simulink model "ArduinoCollectionEEGSimulation"  (R2024b)
settings: Solver=VariableStepAuto  StartTime=0.0  StopTime=10.0  RelTol=1e-3
libraries: dspfdesign x48, arduinolib x16, deeplib x16, audioai x16
settings Model: Creator=dhruva  LastModifiedBy=dhruva

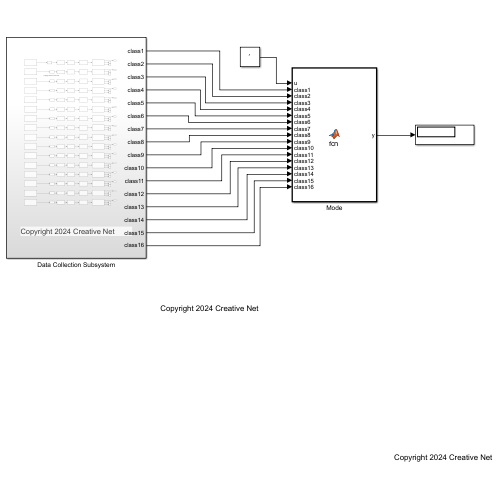
[thumbnail: Simulink's stored preview of the top-level diagram]
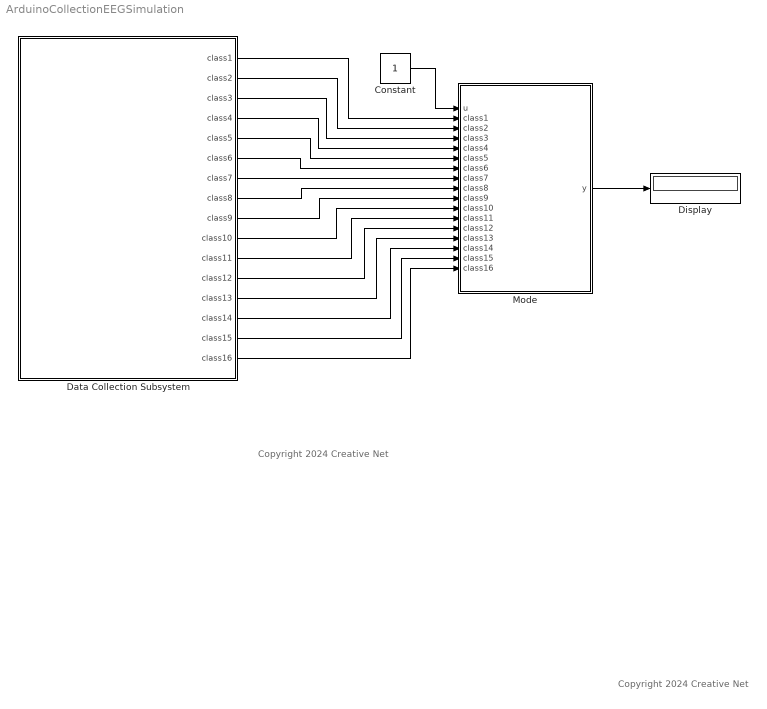
== system ArduinoCollectionEEGSimulation ==
  note: Copyright 2024 Creative Net
  note: Copyright 2024 Creative Net
  Constant : Constant
  Data Collection Subsystem : Subsystem
  Display : Display
  Mode : MATLAB Function  TreatAsAtomicUnit=on
  wires:
  Data Collection Subsystem/1(class1) -> Mode/2(class1)
  Data Collection Subsystem/2(class2) -> Mode/3(class2)
  Data Collection Subsystem/16(class16) -> Mode/17(class16)
  Data Collection Subsystem/15(class15) -> Mode/16(class15)
  Data Collection Subsystem/14(class14) -> Mode/15(class14)
  Data Collection Subsystem/13(class13) -> Mode/14(class13)
  Data Collection Subsystem/12(class12) -> Mode/13(class12)
  Data Collection Subsystem/11(class11) -> Mode/12(class11)
  Data Collection Subsystem/10(class10) -> Mode/11(class10)
  Data Collection Subsystem/3(class3) -> Mode/4(class3)
  Data Collection Subsystem/4(class4) -> Mode/5(class4)
  Data Collection Subsystem/5(class5) -> Mode/6(class5)
  Data Collection Subsystem/6(class6) -> Mode/7(class6)
  Data Collection Subsystem/7(class7) -> Mode/8(class7)
  Data Collection Subsystem/8(class8) -> Mode/9(class8)
  Data Collection Subsystem/9(class9) -> Mode/10(class9)
  Constant/1 -> Mode/1(u)
  Mode/1(y) -> Display/1

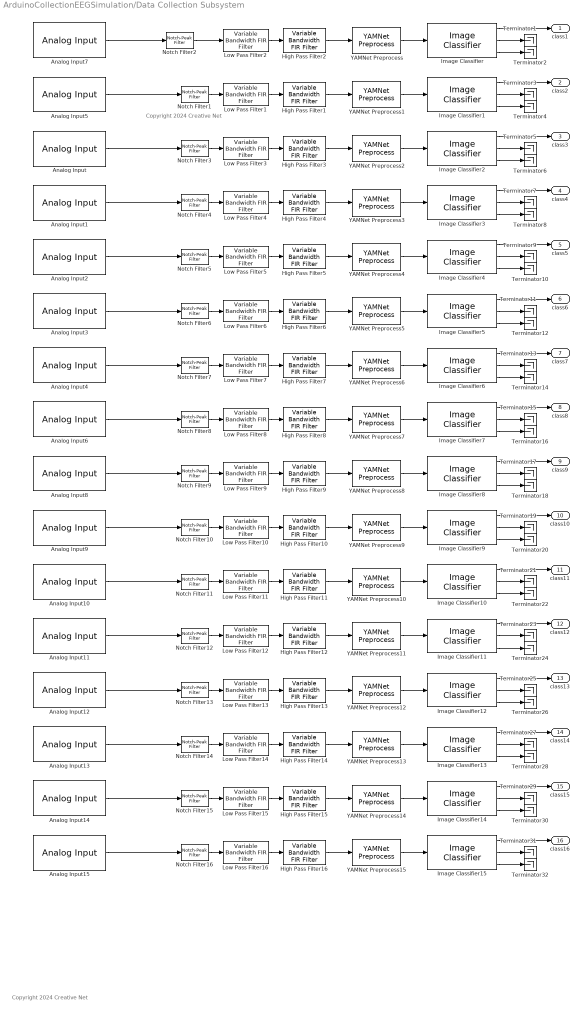
== system ArduinoCollectionEEGSimulation/Data Collection Subsystem ==
  note: Copyright 2024 Creative Net
  note: Copyright 2024 Creative Net
  Analog Input{,1..15} (16 alike) : arduinolib/Analog Input  pinNumber=4  ReadResultsOnly=off  ConversionTriggerSource=Software  ExternalTriggerType=uint32( 0 )  OutputDataType=uint16  EnableConversionCompleteNotify=off  EnableOuputStatus=off  SampleTime=0.008  blockPlatform=arduino
  High Pass Filter{1..16} (16 alike) : dspfdesign/Variable Bandwidth FIR Filter  FilterOrder=30  FilterType=Highpass  CutoffFrequencyPort=off  CutoffFrequency=5  CenterFrequencyPort=off  CenterFrequency=0.5  BandwidthPort=off  Bandwidth=0.3483  Window=Hann  KaiserWindowParameter=.5  SidelobeAttenuation=60  SampleRateMode=Specify on dialog  SampleRate=125  SimulateUsing=Interpreted execution
  Image Classifier{,1..15} (16 alike) : deeplib/Image Classifier  Network=Network from MAT-file  NetworkFunction=squeezenet  NetworkFilePath=D:\projects\Research\Mind Control Bionic Arm\Models\Direct Brainwave Signal\graded learning\model.mat  NetworkClassesVariable=classNames  MiniBatchSize=128  ResizeInput=on  Classification=on  Predictions=on  ForceInterpretedSim=off  PredictMode=All probabilities and labels  K=5
  Low Pass Filter{1..16} (16 alike) : dspfdesign/Variable Bandwidth FIR Filter  FilterOrder=30  FilterType=Lowpass  CutoffFrequencyPort=off  CutoffFrequency=50  CenterFrequencyPort=off  CenterFrequency=0.5  BandwidthPort=off  Bandwidth=0.3483  Window=Hann  KaiserWindowParameter=.5  SidelobeAttenuation=60  SampleRateMode=Specify on dialog  SampleRate=125  SimulateUsing=Interpreted execution
  Notch Filter{1..16} (16 alike) : dspfdesign/Notch-Peak Filter  Specification=Bandwidth and center frequency  BandwidthPort=off  Bandwidth=60  QualityFactorPort=off  QualityFactor=5  CenterFrequencyPort=off  CenterFrequency=30  BandwidthCoefficientPort=off  BandwidthCoefficient=0.72654  CenterFrequencyCoefficientPort=off  CenterFrequencyCoefficient=0  Output=Notch  SampleRateMode=Specify on dialog  SampleRate=125  SimulateUsing=Interpreted execution
  Terminator{1..32} (32 alike) : Terminator
  YAMNet Preprocess{,1..15} (16 alike) : audioai/YAMNet Preprocess  InputSampleRate=16e3  OverlapPercent=50
  class1 : Outport
  class2 : Outport  Port=2
  class3 : Outport  Port=3
  class4 : Outport  Port=4
  class5 : Outport  Port=5
  class6 : Outport  Port=6
  class7 : Outport  Port=7
  class8 : Outport  Port=8
  class9 : Outport  Port=9
  class10 : Outport  Port=10
  class11 : Outport  Port=11
  class12 : Outport  Port=12
  class13 : Outport  Port=13
  class14 : Outport  Port=14
  class15 : Outport  Port=15
  class16 : Outport  Port=16
  wires:
  Notch Filter2/1 -> Low Pass Filter2/1
  Low Pass Filter2/1 -> High Pass Filter2/1
  Analog Input7/1 -> Notch Filter2/1
  Notch Filter1/1 -> Low Pass Filter1/1
  Low Pass Filter1/1 -> High Pass Filter1/1
  Analog Input5/1 -> Notch Filter1/1
  Notch Filter3/1 -> Low Pass Filter3/1
  Low Pass Filter3/1 -> High Pass Filter3/1
  Analog Input/1 -> Notch Filter3/1
  Notch Filter4/1 -> Low Pass Filter4/1
  Low Pass Filter4/1 -> High Pass Filter4/1
  Analog Input1/1 -> Notch Filter4/1
  Notch Filter5/1 -> Low Pass Filter5/1
  Low Pass Filter5/1 -> High Pass Filter5/1
  Analog Input2/1 -> Notch Filter5/1
  Notch Filter6/1 -> Low Pass Filter6/1
  Low Pass Filter6/1 -> High Pass Filter6/1
  Analog Input3/1 -> Notch Filter6/1
  Notch Filter7/1 -> Low Pass Filter7/1
  Low Pass Filter7/1 -> High Pass Filter7/1
  Analog Input4/1 -> Notch Filter7/1
  Notch Filter8/1 -> Low Pass Filter8/1
  Low Pass Filter8/1 -> High Pass Filter8/1
  Analog Input6/1 -> Notch Filter8/1
  Notch Filter9/1 -> Low Pass Filter9/1
  Low Pass Filter9/1 -> High Pass Filter9/1
  Analog Input8/1 -> Notch Filter9/1
  Notch Filter10/1 -> Low Pass Filter10/1
  Low Pass Filter10/1 -> High Pass Filter10/1
  Analog Input9/1 -> Notch Filter10/1
  Notch Filter11/1 -> Low Pass Filter11/1
  Low Pass Filter11/1 -> High Pass Filter11/1
  Analog Input10/1 -> Notch Filter11/1
  Low Pass Filter12/1 -> High Pass Filter12/1
  Notch Filter12/1 -> Low Pass Filter12/1
  Analog Input11/1 -> Notch Filter12/1
  Low Pass Filter13/1 -> High Pass Filter13/1
  Notch Filter13/1 -> Low Pass Filter13/1
  Low Pass Filter14/1 -> High Pass Filter14/1
  Notch Filter14/1 -> Low Pass Filter14/1
  Analog Input13/1 -> Notch Filter14/1
  Analog Input12/1 -> Notch Filter13/1
  Notch Filter15/1 -> Low Pass Filter15/1
  Low Pass Filter15/1 -> High Pass Filter15/1
  Analog Input14/1 -> Notch Filter15/1
  Notch Filter16/1 -> Low Pass Filter16/1
  Low Pass Filter16/1 -> High Pass Filter16/1
  Analog Input15/1 -> Notch Filter16/1
  High Pass Filter2/1 -> YAMNet Preprocess/1
  YAMNet Preprocess/1 -> Image Classifier/1
  Image Classifier/1 -> class1/1
  Image Classifier/2 -> Terminator1/1
  Image Classifier/3 -> Terminator2/1
  YAMNet Preprocess1/1 -> Image Classifier1/1
  Image Classifier1/3 -> Terminator4/1
  Image Classifier1/2 -> Terminator3/1
  High Pass Filter1/1 -> YAMNet Preprocess1/1
  Image Classifier1/1 -> class2/1
  Image Classifier2/2 -> Terminator5/1
  Image Classifier2/3 -> Terminator6/1
  YAMNet Preprocess2/1 -> Image Classifier2/1
  Image Classifier2/1 -> class3/1
  High Pass Filter3/1 -> YAMNet Preprocess2/1
  Image Classifier3/2 -> Terminator7/1
  Image Classifier3/3 -> Terminator8/1
  YAMNet Preprocess3/1 -> Image Classifier3/1
  High Pass Filter4/1 -> YAMNet Preprocess3/1
  Image Classifier3/1 -> class4/1
  Image Classifier4/2 -> Terminator9/1
  Image Classifier4/3 -> Terminator10/1
  YAMNet Preprocess4/1 -> Image Classifier4/1
  High Pass Filter5/1 -> YAMNet Preprocess4/1
  Image Classifier4/1 -> class5/1
  Image Classifier5/2 -> Terminator11/1
  Image Classifier5/3 -> Terminator12/1
  YAMNet Preprocess5/1 -> Image Classifier5/1
  High Pass Filter6/1 -> YAMNet Preprocess5/1
  Image Classifier5/1 -> class6/1
  Image Classifier6/2 -> Terminator13/1
  Image Classifier6/3 -> Terminator14/1
  YAMNet Preprocess6/1 -> Image Classifier6/1
  High Pass Filter7/1 -> YAMNet Preprocess6/1
  Image Classifier6/1 -> class7/1
  Image Classifier7/2 -> Terminator15/1
  Image Classifier7/3 -> Terminator16/1
  YAMNet Preprocess7/1 -> Image Classifier7/1
  High Pass Filter8/1 -> YAMNet Preprocess7/1
  Image Classifier7/1 -> class8/1
  Image Classifier8/2 -> Terminator17/1
  Image Classifier8/3 -> Terminator18/1
  YAMNet Preprocess8/1 -> Image Classifier8/1
  High Pass Filter9/1 -> YAMNet Preprocess8/1
  Image Classifier8/1 -> class9/1
  Image Classifier9/2 -> Terminator19/1
  Image Classifier9/3 -> Terminator20/1
  YAMNet Preprocess9/1 -> Image Classifier9/1
  High Pass Filter10/1 -> YAMNet Preprocess9/1
  Image Classifier9/1 -> class10/1
  Image Classifier10/2 -> Terminator21/1
  Image Classifier10/3 -> Terminator22/1
  YAMNet Preprocess10/1 -> Image Classifier10/1
  High Pass Filter11/1 -> YAMNet Preprocess10/1
  Image Classifier10/1 -> class11/1
  Image Classifier11/2 -> Terminator23/1
  Image Classifier11/3 -> Terminator24/1
  YAMNet Preprocess11/1 -> Image Classifier11/1
  Image Classifier11/1 -> class12/1
  High Pass Filter12/1 -> YAMNet Preprocess11/1
  Image Classifier12/2 -> Terminator25/1
  Image Classifier12/3 -> Terminator26/1
  YAMNet Preprocess12/1 -> Image Classifier12/1
  High Pass Filter13/1 -> YAMNet Preprocess12/1
  Image Classifier12/1 -> class13/1
  Image Classifier13/2 -> Terminator27/1
  Image Classifier13/3 -> Terminator28/1
  YAMNet Preprocess13/1 -> Image Classifier13/1
  Image Classifier13/1 -> class14/1
  High Pass Filter14/1 -> YAMNet Preprocess13/1
  Image Classifier14/2 -> Terminator29/1
  Image Classifier14/3 -> Terminator30/1
  YAMNet Preprocess14/1 -> Image Classifier14/1
  High Pass Filter15/1 -> YAMNet Preprocess14/1
  Image Classifier14/1 -> class15/1
  Image Classifier15/2 -> Terminator31/1
  Image Classifier15/3 -> Terminator32/1
  YAMNet Preprocess15/1 -> Image Classifier15/1
  High Pass Filter16/1 -> YAMNet Preprocess15/1
  Image Classifier15/1 -> class16/1

== matlab function ArduinoCollectionEEGSimulation/Mode ==
  data: u input; y output; class1 input; class2 input; class3 input; class4 input; class5 input; class6 input; class7 input; class8 input; class9 input; class10 input; class11 input; class12 input; class13 input; class14 input; class15 input; class16 input
function y = fcn(u,class1, class2, class3, class4, class5, class6, class7, class8, class9, class10, class11, class12, class13, class14, class15, class16)
y = u;
y(1) = class1;
y(2) = class2;
y(3) = class3;
y(4) = class4;
y(5) = class5;
y(6) = class6;
y(7) = class7;
y(8) = class8;
y(9) = class9;
y(10) = class10;
y(11) = class11;
y(12) = class12;
y(13) = class13;
y(14) = class14;
y(15) = class15;
y(16) = class16;

y = mode(y);
